simulink model "test"  (Simulink 7.3)
settings: Solver=ode45  StartTime=0.0  StopTime=10  RelTol=1e-3
libraries: simulink x1
settings Model: Creator=Sainquake Notebook  LastModifiedBy=Sainquake Notebook

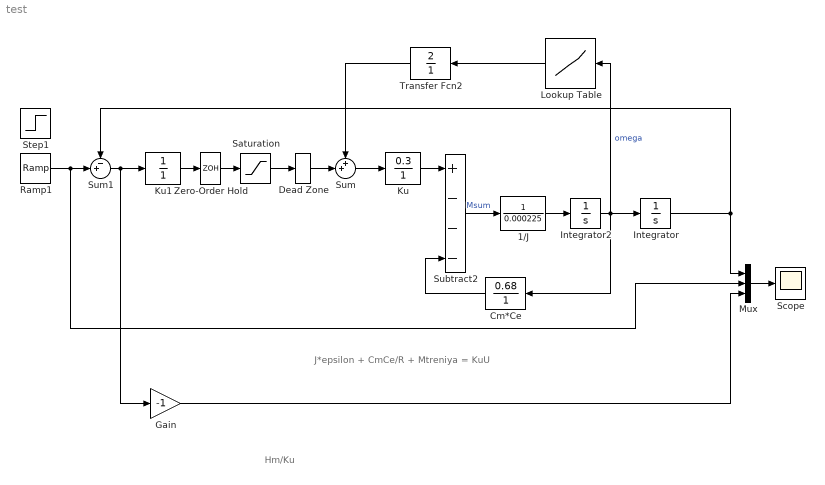
== system test ==
  note: J*epsilon + CmCe/R + Mtreniya = KuU
  note: Hm/Ku
  1/J : TransferFcn  Denominator=0.000225
  Cm*Ce : TransferFcn  Numerator=[0.68]  Denominator=[ 1]
  Dead Zone : DeadZone  SaturateOnIntegerOverflow=on
  Gain : Gain  Gain=-1  ParameterDataType=fixdt(1, 16)  ParameterScaling=2^0  OutDataType=fixdt(1, 16)  OutScaling=2^0
  Integrator : Integrator
  Integrator2 : Integrator
  Ku : TransferFcn  Numerator=0.3  Denominator=[ 1 ]
  Ku1 : TransferFcn  Numerator=1  Denominator=[ 1 ]
  Lookup Table : Lookup  InputValues=[-5:5]  Table=tanh(10*[-5:5])  OutDataType=fixdt(1, 16)  OutScaling=2^0
  Mux : Mux  Inputs=3
  Ramp1 : simulink/Sources/Ramp  SystemSampleTime=-1  slope=-1  start=0  X0=0
  Saturation : Saturate  UpperLimit=10  LowerLimit=-10
  Scope : Scope
      settings: MaxDataPoints=50000
  Step1 : Step  SampleTime=0
  Subtract2 : Sum  Inputs=+---
  Sum : Sum  Inputs=++|  OutDataType=fixdt(1, 16)  OutScaling=2^0
  Sum1 : Sum  Inputs=-+|  OutDataType=fixdt(1, 16)  OutScaling=2^0
  Transfer Fcn2 : TransferFcn  Numerator=2  Denominator=[ 1 ]
  Zero-Order Hold : ZeroOrderHold  SampleTime=1/1000
  wires:
  Subtract2/1 -> 1/J/1  "Msum"
  Integrator2/1 -> Cm*Ce/1, Integrator/1, Lookup Table/1  "omega"
  1/J/1 -> Integrator2/1
  Cm*Ce/1 -> Subtract2/4
  Sum1/1 -> Gain/1, Ku1/1
  Mux/1 -> Scope/1
  Zero-Order Hold/1 -> Saturation/1
  Ramp1/1 -> Sum1/2, Mux/2
  Integrator/1 -> Mux/1, Sum1/1
  Gain/1 -> Mux/3
  Ku/1 -> Subtract2/1
  Ku1/1 -> Zero-Order Hold/1
  Saturation/1 -> Dead Zone/1
  Sum/1 -> Ku/1
  Lookup Table/1 -> Transfer Fcn2/1
  Dead Zone/1 -> Sum/2
  Transfer Fcn2/1 -> Sum/1
